simulink model "DC_motor_KichTu_DocLap"  (R2019a)
settings: Solver=VariableStepAuto  StartTime=0.0  StopTime=10.0  RelTol=1e-3
libraries: powerlib x4
settings Model: Creator=Admin  LastModifiedBy=Admin

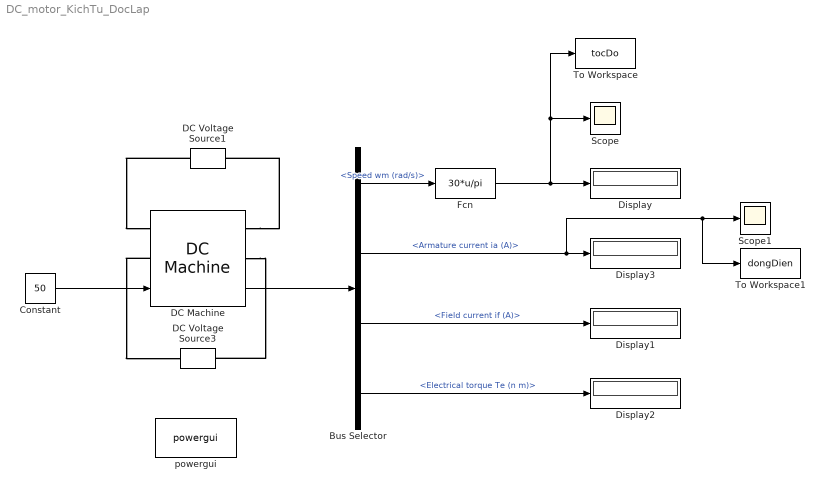
== system DC_motor_KichTu_DocLap ==
  Bus Selector : BusSelector  OutputSignals=Speed wm (rad/s),Armature current ia (A),Field current if (A),Electrical torque Te (n m)
  Constant : Constant  Value=50
  DC Machine : powerlib/Machines/DC Machine  PresetModel=03: 5HP 500V 1750RPM Field:300V  MechanicalLoad=Torque TL  FieldType=Wound  ShowDetailedParameters=on  MeasurementBus=off  RLa=[11.2 0.1215]  RLf=[281.3 156]  Laf=1.976  MachineConstant=Torque constant (N.m/A)  Ke=1.8  Kt=1.8  J=0.02215  Bm=0.002953  Tf=0.5161  w0=1  Ifinit=1  TsPowergui=0  TsBlock=-1
      settings: SourceProductName=Simscape Electrical
  DC Voltage Source1 : powerlib/Electrical Sources/DC Voltage Source  Amplitude=300  Measurements=None
      settings: SourceProductName=Simscape Electrical
  DC Voltage Source3 : powerlib/Electrical Sources/DC Voltage Source  Amplitude=500  Measurements=None
      settings: SourceProductName=Simscape Electrical
  Display{,1..3} (4 alike) : Display
  Fcn : Fcn  Expr=30*u/pi
  Scope : Scope
  Scope1 : Scope
  To Workspace : ToWorkspace  VariableName=tocDo  SaveFormat=Timeseries  SampleTime=-1
  To Workspace1 : ToWorkspace  VariableName=dongDien  SaveFormat=Timeseries  SampleTime=-1
  powergui : powerlib/powergui  Priority=1  SimulationMode=Continuous  SampleTime=50e-6  frequency=60  Iterations=50  frequencyindice=0  Pbase=100e6  ErrMax=1e-4  UnitsV=kV  UnitsW=MW  buscounter=0  FunctionMessages=off  echomessages=off  EnableUseOfTLC=off  CurrentSourceSwitches=off  DisableSnubberDevices=off  DisableRonSwitches=off  DisableVfSwitches=off  DisplayEquations=off  AutomaticDiscreteSolvers=off  SolverType=Tustin/Backward Euler (TBE)  Interpol=off  ExternalGateDelay=off  methode=off  Ts=100  x0status=blocks  SPID=on  SwTol=0  HookPort=off  NonlinearTolerance=0  nMaxIteration=15  ContinueOnMaxIteration=off  RestoreLinks=warning  ResistiveCurrentMeasurement=off  Frange=[0:2:500]  Ylog=off  Xlog=on  ShowGrid=off  save=off  variable=ZData  structure=0  ZoomFFT=off  StartTime=0.0  cycles=1  DisplayStyle=1  fundamental=60  FreqAxis=off  MaxFrequency=1000  frequencyindicesteady=1  RmsSteady=1  display=off
      settings: SourceProductName=Simscape Electrical
  wires:
  Fcn/1 -> To Workspace/1, Scope/1, Display/1
  Constant/1 -> DC Machine/1
  Bus Selector/3 -> Display1/1  "<Field current if (A)>"
  Bus Selector/1 -> Fcn/1  "<Speed wm (rad/s)>"
  Bus Selector/4 -> Display2/1  "<Electrical torque Te (n m)>"
  Bus Selector/2 -> To Workspace1/1, Scope1/1, Display3/1  "<Armature current ia (A)>"
  DC Machine/1 -> Bus Selector/1
  connections:
  DC Voltage Source1/RConn1 -- DC Machine/LConn2
  DC Machine/RConn2 -- DC Voltage Source1/LConn1
  DC Machine/RConn1 -- DC Voltage Source3/LConn1
  DC Machine/LConn1 -- DC Voltage Source3/RConn1
